simulink model "EventAction"  (R2020b)
settings: Solver=VariableStepAuto  StartTime=0.0  StopTime=10.0  RelTol=1e-3
settings Model: Creator=apple  LastModifiedBy=apple

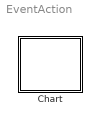
== system EventAction ==
  Chart : Stateflow chart  TreatAsAtomicUnit=on

== stateflow chart EventAction/Chart ==
  state A
    en:fprintf("Entry A");
    du:fprintf("During A");
    ex:fprintf("Exit A");
    state A1
      en:fprintf("Entry A1");
      du:fprintf("During A1");
      ex:fprintf("Exit A1");
    state A2
      en:fprintf("Entry A2");
      du:fprintf("During A2");
      ex:fprintf("Exit A2");
    (default) -> A1
    A1 -> A2 : E_one
    A2 -> A1 : E_two
  state B
    en:fprintf("Entry B");
    du:fprintf("During B");
    ex:fprintf("Exit B");
  (default) -> A
  A -> B : E_four
  events: E_four local FUNCTION_CALL_EVENT; E_one local FUNCTION_CALL_EVENT; E_two local FUNCTION_CALL_EVENT
